simulink model "SistemaCompleto_PMSM"  (R2023b)
settings: Solver=VariableStepAuto  StartTime=0.0  StopTime=2  RelTol=1e-3
PostLoadFcn:
  | parametros_sistema_completo
  | run("parametros_sistema_completo.mlx")
values from neighbouring files (symbols this model uses):
  a_cu = 3.9e-3    (= 0.0039)    [parametros_sistema_completo.m]    (also in workspace_params.mat)
  A_i = [0,  1,                          0 ... (first row only)    [analisis_estabilidad_LA.m]
  b_eq = params.b_total    [calcular_matriz_AO.m]    (also in calculo_incertidumbre_y_control.m = b_m + b_l/(r^2); parametros_sistema_completo.m = 2.19444444444e-05; workspace_params.mat = 2.19444444444e-05)
  C_ts = C_ts * (1 + tol_pct)    [calculo_incertidumbre_y_control.m]    (also in parametros_sistema_completo.m = 0.818; workspace_params.mat = 0.818)
  g = 9.80665    [parametros_sistema_completo.m]    (also in workspace_params.mat)
  J_eq = params.J_total    [calcular_matriz_AO.m]    (also in calculo_incertidumbre_y_control.m = J_m + J_l/r^2; parametros_sistema_completo.m = 1.97847222222e-05; workspace_params.mat = 3.28055555556e-05)
  k_l = m*l_cm + m_l*l_l    [calculo_incertidumbre_y_control.m]    (also in parametros_sistema_completo.m = 0.25; workspace_params.mat = 0.625)
  L_d = L_d    * (1 - tol_pct)    [calculo_incertidumbre_y_control.m]    (also in parametros_sistema_completo.m = 0.0066; workspace_params.mat = 0.0066)
  L_ls = L_ls   * (1 - tol_pct)    [calculo_incertidumbre_y_control.m]    (also in parametros_sistema_completo.m = 0.0008; workspace_params.mat = 0.0008)
  L_q = L_q    * (1 - tol_pct)    [calculo_incertidumbre_y_control.m]    (also in parametros_sistema_completo.m = 0.0058; workspace_params.mat = 0.0058)
  lambda_r = lambda_r * (1 + tol_pct)    [calculo_incertidumbre_y_control.m]    (also in parametros_sistema_completo.m = 0.016; workspace_params.mat = 0.016)
  P_p = 3    [parametros_sistema_completo.m]    (also in workspace_params.mat)
  params = struct()    [evaluar_migracion_Ids.m]    (also in parametros_sistema_completo.m; workspace_params.mat = )
  r = params.r_red    [calcular_matriz_AO.m]    (also in parametros_sistema_completo.m = 120; workspace_params.mat = 120)
  R_s_sim = R_sREF * (1 + a_cu * (T_s_sim - T_sREF))    [configurar_temperatura_516.m]
  R_sREF = R_sREF * (1 - tol_pct)    [calculo_incertidumbre_y_control.m]    (also in parametros_sistema_completo.m = 1.02; workspace_params.mat = 1.02)
  R_ts_amb = R_ts_amb * (1 - tol_pct)    [calculo_incertidumbre_y_control.m]    (also in parametros_sistema_completo.m = 146.7; workspace_params.mat = 146.7)
  T_amb = 20    [parametros_sistema_completo.m]    (also in workspace_params.mat)
  T_s = x(6)    [modulador_torque_521.m]    (also in simulacion_dinamica_516.m)
  T_sREF = 20    [parametros_sistema_completo.m]    (also in workspace_params.mat)
undefined symbols (not defined in the file or in its folder): A_T, A_theta, A_v, b_a, B_i, B_T, B_theta, B_v, C_i, C_T, C_theta, C_v, consigna_posicion, D_i, D_T, D_theta, D_v, i_ds_inicial, Is_pico, Is_rms_max, Is_rms_nom, K_e_i_m_int, K_e_tita_m, K_e_tita_m_int, K_e_w_m, K_e_w_m_int, K_p0, K_pd, K_pq, K_sa, K_sia, pos_inicial, t_rampa_acel, t_rampa_vel, V_sl_max, x0_ias, x0_ibs, x0_ics, x0_T, x0_theta
libraries: simulink_extras x8, SignalEditorBlockLib x6, eeStairGenerator x4, simulink x1
(part 1 of 7)
settings Model: Creator=Francisco  LastModifiedBy=calde
settings DebuggingCC: UnderspecifiedInitializationDetection=Classic  MergeDetectMultiDrivingBlocksExec=none
settings ModelReferenceCC: PropagateSignalLabelsOutOfModel=off

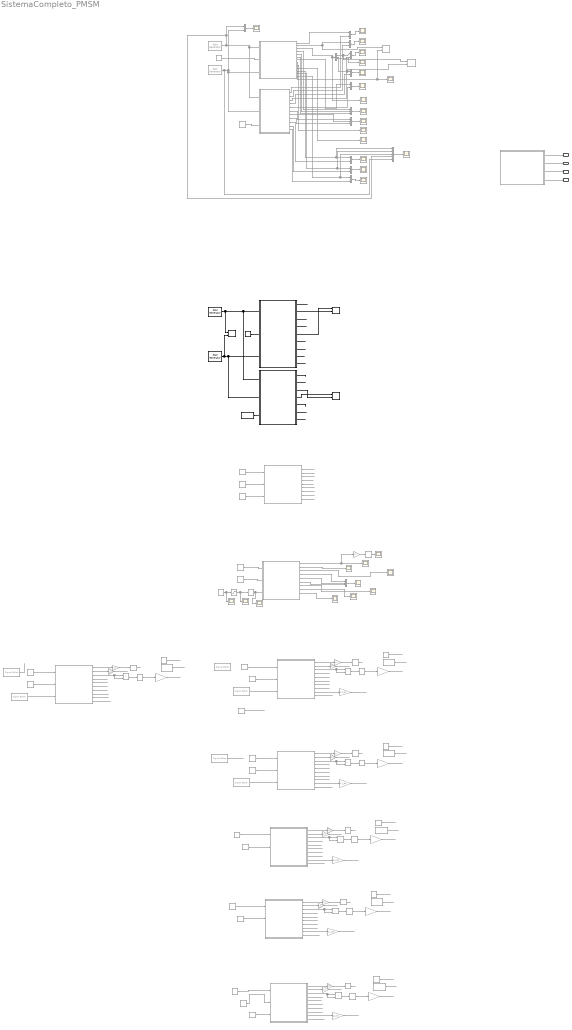
== system SistemaCompleto_PMSM ==
  note: Modelo NL vs LTI Equivalente Aumentado
  note: Consigna de Torque
  note: Consigna de Corriente en eje directo
  note: Consigna de Corriente en eje directo
  note: Consigna de Corriente en eje directo
  note: 5.1.6 Modelo Gobal NL Retroalimentado
      | vs LTI Equivalente Aumentado
  note: Consigna de Corriente en eje directo
  note: Observador de velocidad
      | perfil trapezoidal de velocidad
  note: Consigna de Corriente en eje directo
  note: Consigna de Corriente en eje directo
  note: Consigna de Corriente en eje directo
  note: Consigna de Corriente en eje directo
  note: 5.2.1 Modulador de Torque equivalente
  note: 5.2.2 Controlador externo de movimientos: posición/velocidad
  note: 5.2.3 Observador de velocidad perfil trapezoidal aceleracion
  note: 5.2.7 Controlador Codifiado
  note: 5.2.6 Controlador Discretizado
  note: 5.2.5 Sensores y Acondicionadores de Señal
  note: 5.2.3 Observador de velocidad con accion integral
  Constant{,1..4,6,10..11,14,17,19,23,27} (13 alike) : Constant  Commented=on  Value=0
  Constant{8,12,15,21,25,29} (6 alike) : Constant  Commented=on  Value=Is_rms_max
  Constant{9,13,16,22,26,30} (6 alike) : Constant  Commented=on  Value=Is_rms_nom
  Constant18 : Constant  Commented=on  Value=115
  Constant{7,20,24,28} (4 alike) : Constant  Commented=on  Value=5
  Constant31 : Constant  Commented=on  Value=0.1
  Constant32 : Constant  Commented=on  Value=9.81
  Constant5 : Constant  Value=0
  Degrees to Radians : simulink_extras/Transformations/Degrees to Radians  Commented=on
  Demux : Demux  Commented=on  Outputs=3
  Dot Product{,1..5} (6 alike) : DotProduct  Commented=on  OutDataTypeStr=Inherit: Inherit via internal rule
  Gain{,1,3,5,7,9,11..12,14,16,18,20,22} (13 alike) : Gain  Commented=on  Gain=1/r
  Gain{2,6,10,13,17,21} (6 alike) : Gain  Commented=on  Gain=1/sqrt(2)
  Gain{4,8,15,19,23} (5 alike) : Gain  Commented=on  Gain=1/J_eq
  I_abc : Scope  Commented=on
  I_abc2 : Scope  Commented=on
  I_abc3 : Scope  Commented=on
  I_qds : Scope  Commented=on
  I_qds2 : Scope  Commented=on
  LTI Equivalente Aumentado : Subsystem  Commented=on
  LTI Equivalente Aumentado2 : Subsystem
  LTI Equivalente Nominal : Subsystem  Commented=on
  "Modelo Global " : Subsystem  Commented=on
  Modelo Global NL Controlador modulador de torque : Subsystem  Commented=on
  Modelo Global NL Controlador modulador de torque1 : Subsystem  Commented=on
  Modelo Global NL Controlador modulador de torque3 : Subsystem  Commented=on
  Modelo Global NL Controlador modulador de torque4 : Subsystem  Commented=on
  Modelo Global NL perfil trapezoidal aceleracion : Subsystem  Commented=on
  Modelo Global NL perfil trapezoidal aceleracion y codificado : Subsystem  Commented=on
  Modelo Global NL perfil trapezoidal aceleracion1 : Subsystem  Commented=on
  Modelo Global NL perfil trapezoidal aceleracion2 : Subsystem  Commented=on
  Modelo Global NL Retroalimentado : Subsystem
  Mux{,1..5,8..10} (9 alike) : Mux  Commented=on  Inputs=2
  Mux11 : Mux  Commented=on  Inputs=3
  Mux12 : Mux  Commented=on  Inputs=5
  Mux13 : Mux  Commented=on  Inputs=3
  Mux6 : Mux  Commented=on  Inputs=3
  Radians to Degrees{,1..6} (7 alike) : simulink_extras/Transformations/Radians to Degrees  Commented=on
  Ramp : simulink/Sources/Ramp  Commented=on  slope=300  start=0  InitialOutput=0
  Saturation : Saturate  Commented=on  UpperLimit=135  LowerLimit=0
  Scope1 : Scope  Commented=on
  Scope2 : Scope  Commented=on
  Scope3 : Scope  Commented=on
  Signal Editor : SignalEditorBlockLib/Signal Editor  Commented=on  FileName=C:\Users\calde\OneDrive\Documents\00_INGENIERIA\1_CURSADO\2 2025\AyME\modelado-control-motor-pmsm\Señales y Escenarios\trap_posicion_1.mat  ActiveScenario=TrapezoidalPosicion  ActiveSignal=posicion  IsBus=off  OutputBusObjectStr=Bus: BusObject  SampleTime=0  ZeroCross=off  OutputAfterFinalValue=Setting to zero  Unit=inherit  PreserveSignalName=on  ApplySigPropsToAllScenarios=on  ApplySigPropsToAllSignals=off
  Signal Editor1 : SignalEditorBlockLib/Signal Editor  Commented=on  FileName=C:\Users\calde\OneDrive\Documents\00_INGENIERIA\1_CURSADO\2 2025\AyME\modelado-control-motor-pmsm\Señales\perturbacion_Tld.mat  ActiveScenario=Perturbacion  ActiveSignal=Signal 1  IsBus=off  OutputBusObjectStr=Bus: BusObject  SampleTime=0  Interpolate=off  ZeroCross=off  OutputAfterFinalValue=Setting to zero  Unit=inherit  PreserveSignalName=on  ApplySigPropsToAllScenarios=on  ApplySigPropsToAllSignals=off
  Signal Editor2 : SignalEditorBlockLib/Signal Editor  Commented=on  FileName=D:\05.Estudios\Trabajo Final AyME 2025\modelado-control-motor-pmsm\Señales y Escenarios\trap_posicion_1.mat  ActiveScenario=TrapezoidalPosicion  ActiveSignal=posicion  IsBus=off  OutputBusObjectStr=Bus: BusObject  SampleTime=0  ZeroCross=off  OutputAfterFinalValue=Setting to zero  Unit=inherit  PreserveSignalName=on  ApplySigPropsToAllScenarios=on  ApplySigPropsToAllSignals=off
  Signal Editor3 : SignalEditorBlockLib/Signal Editor  Commented=on  FileName=D:\05.Estudios\Trabajo Final AyME 2025\modelado-control-motor-pmsm\Señales\perturbacion_Tld.mat  ActiveScenario=Perturbacion  ActiveSignal=Signal 1  IsBus=off  OutputBusObjectStr=Bus: BusObject  SampleTime=0  Interpolate=off  ZeroCross=off  OutputAfterFinalValue=Setting to zero  Unit=inherit  PreserveSignalName=on  ApplySigPropsToAllScenarios=on  ApplySigPropsToAllSignals=off
  Signal Editor4 : SignalEditorBlockLib/Signal Editor  Commented=on  FileName=D:\05.Estudios\Trabajo Final AyME 2025\modelado-control-motor-pmsm\Señales y Escenarios\trap_posicion_1.mat  ActiveScenario=TrapezoidalPosicion  ActiveSignal=posicion  IsBus=off  OutputBusObjectStr=Bus: BusObject  SampleTime=0  ZeroCross=off  OutputAfterFinalValue=Setting to zero  Unit=inherit  PreserveSignalName=on  ApplySigPropsToAllScenarios=on  ApplySigPropsToAllSignals=off
  Signal Editor5 : SignalEditorBlockLib/Signal Editor  Commented=on  FileName=D:\05.Estudios\Trabajo Final AyME 2025\modelado-control-motor-pmsm\Señales\perturbacion_Tld.mat  ActiveScenario=Perturbacion  ActiveSignal=Signal 1  IsBus=off  OutputBusObjectStr=Bus: BusObject  SampleTime=0  Interpolate=off  ZeroCross=off  OutputAfterFinalValue=Setting to zero  Unit=inherit  PreserveSignalName=on  ApplySigPropsToAllScenarios=on  ApplySigPropsToAllSignals=off
  Sqrt{,1..5} (6 alike) : Sqrt  Commented=on
  T_amb : Constant  Commented=on  Value=T_amb
  T_amb2 : Constant  Value=T_amb
  T_l : eeStairGenerator/Stair Generator  Commented=on  LabelModeActiveChoice=Discrete  TimeInput=[0 0.3 0.5 0.9 1.3 1.5 1.9]  AmplitudeInput=[0 6.28 -6.28 0 6.28 -6.28 0]  SampleTime=1e-3  RepeatPattern=off  OutDataTypeStr=double
      settings: LibrarySourceBlock=ee_sl_lib/General Control/Stair Generator
  T_l2 : eeStairGenerator/Stair Generator  LabelModeActiveChoice=Discrete  TimeInput=[0 0.3 0.5 0.9 1.3 1.5 1.9]  AmplitudeInput=[0 6.28 -6.28 0 6.28 -6.28 0]  SampleTime=1e-3  RepeatPattern=off  OutDataTypeStr=double
      settings: LibrarySourceBlock=ee_sl_lib/General Control/Stair Generator
  T_m [N.m] : Scope  Commented=on
  T_m [N.m]3 : Scope  Commented=on
  T_m [N.m]4 : Scope  Commented=on
  T_s (vs) : Scope  Commented=on
  T_s(t)1 : Scope  Commented=on
  Torque vs. Velocidad : Record  Commented=on  FileSettingsInternal="{\"entries\":[{\"content\":{\"excelSettings\":{\"content\":{},\"type\":\"Streamout.ExcelSettings\"}},\"type\":\"Streamout.FileSettingStorage\",\"uuid\":\"\"}],\"packageUris\":[\"http:\\/\\/schema.mathworks.com\\/mf0\\/streamout_blocks\\/R2020a\"],\"version\":\"1.0\"}"  Layout=[1 1]  SignalsInternal="{\"entries\":[{\"content\":{},\"type\":\"RecordBlkView.InputSignals\",\"uuid\":\"\"}],\"packageUris\":[\"http:\\/\\/schema.mathworks.com\\/mf0\\/streamout_blocks\\/R2020a\"],\"version\":\"1.0\"}"  VisualizationBindings="{\"xyplotplugin\":{\"info\":[{\"series\":[],\"subplotID\":1}]}}"  CompatibilityTag=XY
  Torque vs. Velocidad2 : Record  FileSettingsInternal="{\"entries\":[{\"content\":{\"excelSettings\":{\"content\":{},\"type\":\"Streamout.ExcelSettings\"}},\"type\":\"Streamout.FileSettingStorage\",\"uuid\":\"\"}],\"packageUris\":[\"http:\\/\\/schema.mathworks.com\\/mf0\\/streamout_blocks\\/R2020a\"],\"version\":\"1.0\"}"  Layout=[1 1]  SignalsInternal="{\"entries\":[{\"content\":{\"signals\":[{\"content\":{\"blockPath\":[],\"dimensions\":[1],\"domain\":\"\",\"lineColor\":\"#d95319\",\"port\":1,\"sid\":[\"\"],\"signalID\":4289,\"signalName\":\"NL T_m [N.m]\"},\"type\":\"RecordBlkView.Signal\",\"uuid\":\"\"},{\"content\":{\"blockPath\":[],\"dimensions\":[1],\"domain\":\"\",\"lineColor\":\"#edb120\",\"port\":2,\"sid\":[\"\"],\"signalID\":4293,\"signalName\":\"NL ω_m [rad\\/s]\"},\"type\":\"RecordBlkView.Signal\",\"uuid\":\"\"}]},\"type\":\"RecordBlkView.InputSignals\",\"uuid\":\"\"}],\"packageUris\":[\"http:\\/\\/schema.mathworks.com\\/mf0\\/streamout_blocks\\/R2020a\"],\"version\":\"1.0\"}"  VisualizationBindings="{\"xyplotplugin\":{\"info\":[{\"series\":[],\"subplotID\":1}]}}"  CompatibilityTag=XY
  V_a : Scope  Commented=on
  V_abc vs V_qs-T_l : Scope  Commented=on
  V_b : Scope  Commented=on
  V_c : Scope  Commented=on
  V_ds : Scope  Commented=on
  V_qs* : eeStairGenerator/Stair Generator  Commented=on  LabelModeActiveChoice=Discrete  TimeInput=[0 0.1 0.7 1.1 1.7]  AmplitudeInput=[0 19.596 0 -19.596 0]  SampleTime=1e-3  RepeatPattern=off  OutDataTypeStr=double
      settings: LibrarySourceBlock=ee_sl_lib/General Control/Stair Generator
  V_qs*2 : eeStairGenerator/Stair Generator  LabelModeActiveChoice=Discrete  TimeInput=[0 0.1 0.7 1.1 1.7]  AmplitudeInput=[0 19.596 0 -19.596 0]  SampleTime=1e-3  RepeatPattern=off  OutDataTypeStr=double
      settings: LibrarySourceBlock=ee_sl_lib/General Control/Stair Generator
  "V_qs, T_l vs t" : Scope  Commented=on
  "V_qs, T_l vs t2" : Record  FileSettingsInternal="{\"entries\":[{\"content\":{\"excelSettings\":{\"content\":{},\"type\":\"Streamout.ExcelSettings\"}},\"type\":\"Streamout.FileSettingStorage\",\"uuid\":\"\"}],\"packageUris\":[\"http:\\/\\/schema.mathworks.com\\/mf0\\/streamout_blocks\\/R2020a\"],\"version\":\"1.0\"}"  Layout=[1 1]  SignalsInternal="{\"entries\":[{\"content\":{\"signals\":[{\"content\":{\"blockPath\":[],\"dimensions\":[1,1],\"domain\":\"\",\"lineColor\":\"#b746ff\",\"lineWidth\":2,\"port\":1,\"sid\":[\"\"],\"signalID\":4297,\"signalName\":\"V_qs*\"},\"type\":\"RecordBlkView.Signal\",\"uuid\":\"\"},{\"content\":{\"blockPath\":[],\"dimensions\":[1,1],\"domain\":\"\",\"lineColor\":\"#64d413\",\"lineWidth\":2,\"port\":2,\"sid\":[\"\"],\"signalID\":4301,\"signalName\":\"T_l\"},\"type\":\"RecordBlkView.Signal\",\"uuid\":\"\"}]},\"type\":\"RecordBlkView.InputSignals\",\"uuid\":\"\"}],\"packageUris\":[\"http:\\/\\/schema.mathworks.com\\/mf0\\/streamout_blocks\\/R2020a\"],\"version\":\"1.0\"}"  VisualizationBindings="{\"xyplotplugin\":{\"info\":[{\"series\":[],\"subplotID\":1}]}}"  CompatibilityTag=XY
  i_0s vs t : Scope  Commented=on
  i_ds vs i_qs : Record  Commented=on  FileSettingsInternal="{\"entries\":[{\"content\":{\"excelSettings\":{\"content\":{},\"type\":\"Streamout.ExcelSettings\"}},\"type\":\"Streamout.FileSettingStorage\",\"uuid\":\"\"}],\"packageUris\":[\"http:\\/\\/schema.mathworks.com\\/mf0\\/streamout_blocks\\/R2020a\"],\"version\":\"1.0\"}"  Layout=[1 1]  SignalsInternal="{\"entries\":[{\"content\":{},\"type\":\"RecordBlkView.InputSignals\",\"uuid\":\"\"}],\"packageUris\":[\"http:\\/\\/schema.mathworks.com\\/mf0\\/streamout_blocks\\/R2020a\"],\"version\":\"1.0\"}"  VisualizationBindings="{\"xyplotplugin\":{\"info\":[{\"series\":[],\"subplotID\":1}]}}"  CompatibilityTag=XY
  i_ds vs i_qs2 : Record  FileSettingsInternal="{\"entries\":[{\"content\":{\"excelSettings\":{\"content\":{},\"type\":\"Streamout.ExcelSettings\"}},\"type\":\"Streamout.FileSettingStorage\",\"uuid\":\"\"}],\"packageUris\":[\"http:\\/\\/schema.mathworks.com\\/mf0\\/streamout_blocks\\/R2020a\"],\"version\":\"1.0\"}"  Layout=[1 1]  SignalsInternal="{\"entries\":[{\"content\":{\"signals\":[{\"content\":{\"blockPath\":[],\"dimensions\":[1],\"domain\":\"\",\"lineColor\":\"#4dbeee\",\"port\":1,\"sid\":[\"\"],\"signalID\":4305,\"signalName\":\"LTI i_ds [A\"},\"type\":\"RecordBlkView.Signal\",\"uuid\":\"\"},{\"content\":{\"blockPath\":[],\"dimensions\":[1],\"domain\":\"\",\"lineColor\":\"#a2142f\",\"port\":2,\"sid\":[\"\"],\"signalID\":4309,\"signalName\":\"LTI i_qs [A]\"},\"type\":\"RecordBlkView.Signal\",\"uuid\":\"\"}]},\"type\":\"RecordBlkView.InputSignals\",\"uuid\":\"\"}],\"packageUris\":[\"http:\\/\\/schema.mathworks.com\\/mf0\\/streamout_blocks\\/R2020a\"],\"version\":\"1.0\"}"  VisualizationBindings="{\"xyplotplugin\":{\"info\":[{\"series\":[],\"subplotID\":1}]}}"  CompatibilityTag=XY
  i_ds vs t : Scope  Commented=on
  i_qs vs t : Scope  Commented=on
  δ [rad] : Scope  Commented=on
  θm(t) vs t : Scope  Commented=on
  θm(t) vs t 2 : Scope  Commented=on
  θm(t) vs t 3 : Scope  Commented=on
  ωm(t) vs t : Scope  Commented=on
  ωm(t) vs t2 : Scope  Commented=on
  θ_m : Outport
  ω_m : Outport  Port=2
  i_qs : Outport  Port=3
  T_s : Outport  Port=4
  wires:
  LTI Equivalente Nominal/1(θ_m) -> θ_m/1
  LTI Equivalente Nominal/2(ω_m) -> ω_m/1
  LTI Equivalente Nominal/3(i_qs) -> i_qs/1
  LTI Equivalente Nominal/4(T_s) -> T_s/1
  V_qs*/1 -> Mux12/4, Mux5/1, LTI Equivalente Aumentado/1(v_qs), "Modelo Global "/1(V_qs*[V])
  T_l/1 -> Mux12/5, LTI Equivalente Aumentado/2(T_ld), "Modelo Global "/3(Tld [N.m]), Mux5/2
  T_amb/1 -> LTI Equivalente Aumentado/3(T_amb)
  Constant/1 -> "Modelo Global "/2(V_ds*[V])
  LTI Equivalente Aumentado/1(θ_m [rad]) -> Mux/2
  Mux/1 -> θm(t) vs t/1
  "Modelo Global "/1(θ_m [rad]) -> Mux/1
  "Modelo Global "/3(I_qd0s [A]) -> I_qds/1, Demux/1
  Demux/1 -> Mux3/1, i_ds vs i_qs/1
  Demux/2 -> i_ds vs i_qs/2, Mux2/1
  LTI Equivalente Aumentado/3(i_qs [A]) -> Mux3/2
  LTI Equivalente Aumentado/4(i_ds [A]) -> Mux2/2
  Mux3/1 -> i_qs vs t/1
  Mux2/1 -> i_ds vs t/1
  "Modelo Global "/7(T_s [°C]) -> Mux1/1
  LTI Equivalente Aumentado/5(T_s [°C]) -> Mux1/2
  Mux1/1 -> T_s (vs)/1
  Mux4/1 -> ωm(t) vs t/1
  "Modelo Global "/2(ω_m [rad/s]) -> Mux4/1, Torque vs. Velocidad/1  "ω_m [rad/s]"
  LTI Equivalente Aumentado/2(ω_m [rad/s]) -> Mux4/2
  "Modelo Global "/8(T_m [N.m]) -> Torque vs. Velocidad/2, T_m [N.m]/1  "T_m [N.m]"
  Mux5/1 -> "V_qs, T_l vs t"/1
  Mux6/1 -> I_abc/1
  "Modelo Global "/4(I_a [A]) -> Mux6/1
  "Modelo Global "/5(I_b [A]) -> Mux6/2
  "Modelo Global "/6(I_c [A]) -> Mux6/3
  Demux/3 -> i_0s vs t/1
  "Modelo Global "/9(δ [rad]) -> δ [rad]/1  "δ [rad]"
  "Modelo Global "/10(V_ds[V]) -> V_ds/1
  Mux10/1 -> V_c/1
  Mux9/1 -> V_b/1
  Mux8/1 -> V_a/1
  LTI Equivalente Aumentado/9(V_a) -> Mux8/2
  LTI Equivalente Aumentado/10(V_b) -> Mux9/2
  LTI Equivalente Aumentado/11(V_c) -> Mux10/2
  "Modelo Global "/11(V_a) -> Mux12/1, Mux8/1
  "Modelo Global "/12(V_b) -> Mux12/2, Mux9/1
  "Modelo Global "/13(V_c) -> Mux12/3, Mux10/1
  Mux11/1 -> I_abc2/1
  LTI Equivalente Aumentado/6(I_a [A]) -> Mux11/1
  LTI Equivalente Aumentado/7(I_b [A]) -> Mux11/2
  LTI Equivalente Aumentado/8(I_c [A]) -> Mux11/3
  Mux12/1 -> V_abc vs V_qs-T_l/1
  Modelo Global NL Controlador modulador de torque/5(I_b [A]) -> ?  "I_b [A]"
  Modelo Global NL Controlador modulador de torque/3(I_qd0s [A]) -> ?  "I_qd0s [A]"
  Constant2/1 -> Modelo Global NL Controlador modulador de torque/2(i_ds*)
  Modelo Global NL Controlador modulador de torque/6(I_c [A]) -> ?  "I_c [A]"
  Modelo Global NL Controlador modulador de torque/7(T_s [°C]) -> ?  "T_s [°C]"
  Modelo Global NL Controlador modulador de torque/1(θm(t) [rad]) -> ?  "θm(t) [rad]"
  Modelo Global NL Controlador modulador de torque/4(I_a [A]) -> ?  "I_a [A]"
  Constant1/1 -> Modelo Global NL Controlador modulador de torque/1(Tld [N.m])
  Modelo Global NL Controlador modulador de torque/2(ωm(t) [rad/s]) -> ?  "ωm(t) [rad/s]"
  Modelo Global NL Controlador modulador de torque/8(T_m [N.m]) -> ?  "T_m [N.m]"
  Constant31/1 -> Modelo Global NL Controlador modulador de torque/3(T_m*[N.m])  "T_m*[N.m]"
  Modelo Global NL Controlador modulador de torque1/8(T_m [N.m]) -> T_m [N.m]3/1  "T_m [N.m]"
  Modelo Global NL Controlador modulador de torque1/4(I_a [A]) -> Mux13/1
  Modelo Global NL Controlador modulador de torque1/3(I_qd0s [A]) -> I_qds2/1
  Modelo Global NL Controlador modulador de torque1/6(I_c [A]) -> Mux13/3
  Modelo Global NL Controlador modulador de torque1/1(θm(t) [rad]) -> Gain/1, θm(t) vs t 2/1  "θm(t) [rad]"
  Constant4/1 -> Modelo Global NL Controlador modulador de torque1/2(i_ds*)
  Modelo Global NL Controlador modulador de torque1/5(I_b [A]) -> Mux13/2
  Modelo Global NL Controlador modulador de torque1/2(ωm(t) [rad/s]) -> ωm(t) vs t2/1  "ωm(t) [rad/s]"
  Constant3/1 -> Modelo Global NL Controlador modulador de torque1/1(Tld [N.m])
  Mux13/1 -> I_abc3/1
  Modelo Global NL Controlador modulador de torque1/7(T_s [°C]) -> T_s(t)1/1
  Degrees to Radians/1 -> Scope3/1, Modelo Global NL Controlador modulador de torque1/3(θl*(t))
  Saturation/1 -> Scope1/1, Degrees to Radians/1
  Ramp/1 -> Scope2/1, Saturation/1
  Gain/1 -> Radians to Degrees/1
  Radians to Degrees/1 -> θm(t) vs t 3/1
  Modelo Global NL Controlador modulador de torque1/9(T_neto) -> T_m [N.m]4/1  "T_neto [N.m]"
  Radians to Degrees1/1 -> ?
  Modelo Global NL perfil trapezoidal aceleracion/4(I_a [A]) -> ?  "I_a [A]"
  Modelo Global NL perfil trapezoidal aceleracion/9(T_neto) -> Gain4/1  "T_neto [N.m]"
  Modelo Global NL perfil trapezoidal aceleracion/1(θm(t) [rad]) -> Gain1/1  "θm(t) [rad]"
  Gain1/1 -> Radians to Degrees1/1  "θl(t) [rad]"
  Modelo Global NL perfil trapezoidal aceleracion/5(I_b [A]) -> ?  "I_b [A]"
  Modelo Global NL perfil trapezoidal aceleracion/6(I_c [A]) -> ?  "I_c [A]"
  Modelo Global NL perfil trapezoidal aceleracion/7(T_s [°C]) -> ?  "T_s [°C]"
  Constant6/1 -> Modelo Global NL perfil trapezoidal aceleracion/2(i_ds*)
  Modelo Global NL perfil trapezoidal aceleracion/2(ω~_m(t) [rad/s]) -> Gain3/1  "ω~_m(t) [rad/s]"
  Modelo Global NL perfil trapezoidal aceleracion/8(T_m [N.m]) -> ?  "T_m [N.m]"
  Signal Editor/1 -> Modelo Global NL perfil trapezoidal aceleracion/3(θl*(t))  "θl*(t) [rad]"
  Gain2/1 -> ?  "I_rms"
  Modelo Global NL perfil trapezoidal aceleracion/3(I_qd0s [A]) -> Dot Product/2, Dot Product/1  "I_qd0s [A]"
  Dot Product/1 -> Sqrt/1
  Sqrt/1 -> Gain2/1  "I_stator"
  Constant8/1 -> ?  "I_rms_max"
  Constant9/1 -> ?  "I_rms_nom"
  Modelo Global NL Retroalimentado/3(I_qd0s [A]) -> ?  "NL I_qd0s [A]"
  Modelo Global NL Retroalimentado/1(θ_m [rad]) -> ?  "NL θ_m [rad]"
  LTI Equivalente Aumentado2/1(θ_m [rad]) -> ?  "LTI θ_m [rad]"
  Modelo Global NL Retroalimentado/4(T_s [°C]) -> ?  "NL T_s [°C]"
  Modelo Global NL Retroalimentado/6(δ [deg]) -> ?  "NL δ [deg]"
  Modelo Global NL Retroalimentado/7(V_ds[V]) -> ?  "NL V_ds[V]"
  Modelo Global NL Retroalimentado/9(V_abc [V]) -> ?  "NL V_abc [V]"
  LTI Equivalente Aumentado2/6(I_abc [A]) -> ?  "LTI I_abc [A]"
  Modelo Global NL Retroalimentado/8(I_abc [A]) -> ?  "NL I_abc [A]"
  LTI Equivalente Aumentado2/7(V_abc [V]) -> ?  "LTI V_abc [V]"
  LTI Equivalente Aumentado2/5(T_s [°C]) -> ?  "LTI T_s [°C]"
  LTI Equivalente Aumentado2/4(i_ds [A]) -> i_ds vs i_qs2/1  "LTI i_ds [A"
  T_l2/1 -> Modelo Global NL Retroalimentado/3(Tld [N.m]), LTI Equivalente Aumentado2/2(T_ld), "V_qs, T_l vs t2"/2  "T_l"
  Constant5/1 -> Modelo Global NL Retroalimentado/2(V_ds*[V])  "v_ds*"
  LTI Equivalente Aumentado2/3(i_qs [A]) -> i_ds vs i_qs2/2  "LTI i_qs [A]"
  LTI Equivalente Aumentado2/2(ω_m [rad/s]) -> ?  "LTI ω_m [rad/s]"
  V_qs*2/1 -> Modelo Global NL Retroalimentado/1(V_qs*[V]), LTI Equivalente Aumentado2/1(v_qs), "V_qs, T_l vs t2"/1  "V_qs*"
  Modelo Global NL Retroalimentado/2(ω_m [rad/s]) -> Torque vs. Velocidad2/2  "NL ω_m [rad/s]"
  T_amb2/1 -> LTI Equivalente Aumentado2/3(T_amb)
  Modelo Global NL Retroalimentado/5(T_m [N.m]) -> Torque vs. Velocidad2/1  "NL T_m [N.m]"
  Constant7/1 -> Modelo Global NL perfil trapezoidal aceleracion/1(Tld [N.m])  "Tld [N.m]"
  Gain3/1 -> ?  "ω~_l(t) [rad/s]"
  Modelo Global NL perfil trapezoidal aceleracion/10(θl* [rad]) -> ?  "Trayectoria Pos"
  Gain4/1 -> ?  "Aceleracion"
  Signal Editor3/1 -> ?  "Tld [N.m]"
  Gain8/1 -> ?  "Aceleracion"
  Sqrt1/1 -> Gain6/1  "I_stator"
  Modelo Global NL Controlador modulador de torque3/2(ω~_m(t) [rad/s]) -> Gain7/1  "ω~_m(t) [rad/s]"
  Dot Product1/1 -> Sqrt1/1
  Modelo Global NL Controlador modulador de torque3/1(θm(t) [rad]) -> Gain5/1  "θm(t) [rad]"
  Gain5/1 -> Radians to Degrees2/1  "θl(t) [rad]"
  Constant11/1 -> Modelo Global NL Controlador modulador de torque3/1(Tld [N.m])
  Modelo Global NL Controlador modulador de torque3/9(T_neto) -> Gain8/1  "T_neto [N.m]"
  Modelo Global NL Controlador modulador de torque3/3(I_qd0s [A]) -> Dot Product1/2, Dot Product1/1  "I_qd0s [A]"
  Gain7/1 -> ?  "ω~_l(t) [rad/s]"
  Signal Editor2/1 -> Modelo Global NL Controlador modulador de torque3/3(θl*(t))  "θl*(t) [rad]"
  Constant10/1 -> Modelo Global NL Controlador modulador de torque3/2(i_ds*)
  Radians to Degrees2/1 -> ?
  Modelo Global NL Controlador modulador de torque3/4(I_a [A]) -> ?  "I_a [A]"
  Modelo Global NL Controlador modulador de torque3/8(T_m [N.m]) -> ?  "T_m [N.m]"
  Gain6/1 -> ?  "I_rms"
  Constant12/1 -> ?  "I_rms_max"
  Modelo Global NL Controlador modulador de torque3/5(I_b [A]) -> ?  "I_b [A]"
  Modelo Global NL Controlador modulador de torque3/6(I_c [A]) -> ?  "I_c [A]"
  Modelo Global NL Controlador modulador de torque3/10(θl* [rad]) -> ?  "Trayectoria Pos"
  Modelo Global NL Controlador modulador de torque3/7(T_s [°C]) -> ?  "T_s [°C]"
  Constant13/1 -> ?  "I_rms_nom"
  Gain9/1 -> Radians to Degrees3/1  "θl(t) [rad]"
  Modelo Global NL Controlador modulador de torque4/4(I_a [A]) -> ?  "I_a [A]"
  Modelo Global NL Controlador modulador de torque4/5(I_b [A]) -> ?  "I_b [A]"
  Radians to Degrees3/1 -> ?
  Modelo Global NL Controlador modulador de torque4/6(I_c [A]) -> ?  "I_c [A]"
  Modelo Global NL Controlador modulador de torque4/8(T_m [N.m]) -> ?  "T_m [N.m]"
  Modelo Global NL Controlador modulador de torque4/7(T_s [°C]) -> ?  "T_s [°C]"
  Constant15/1 -> ?  "I_rms_max"
  Constant16/1 -> ?  "I_rms_nom"
  Gain11/1 -> ?  "ω~_l(t) [rad/s]"
  Modelo Global NL Controlador modulador de torque4/10(θm* [rad]) -> ?  "Trayectoria Pos"
  Modelo Global NL Controlador modulador de torque4/3(I_qd0s [A]) -> Dot Product2/2, Dot Product2/1  "I_qd0s [A]"
  Sqrt2/1 -> Gain10/1  "I_stator"
  Signal Editor4/1 -> Modelo Global NL Controlador modulador de torque4/3(θl*(t))  "θl*(t) [rad]"
  Dot Product2/1 -> Sqrt2/1
  Gain10/1 -> ?  "I_rms"
  Signal Editor5/1 -> ?  "Tld [N.m]"
  Constant14/1 -> Modelo Global NL Controlador modulador de torque4/2(i_ds*)
  Modelo Global NL Controlador modulador de torque4/9(T_neto) -> ?  "T_neto [N.m]"
  Modelo Global NL Controlador modulador de torque4/2(ω~_m(t) [rad/s]) -> Gain11/1  "ω~_m(t) [rad/s]"
  Modelo Global NL Controlador modulador de torque4/1(θm(t) [rad]) -> Gain9/1  "θm(t) [rad]"
  Constant17/1 -> Modelo Global NL Controlador modulador de torque4/1(Tld [N.m])
  Constant18/1 -> ?  "Ts°_max"
  Constant20/1 -> Modelo Global NL perfil trapezoidal aceleracion1/1(Tld [N.m])  "Tld [N.m]"
  ? -> Modelo Global NL perfil trapezoidal aceleracion1/3(θl*(t))  "θl*(t) [rad]"
  Modelo Global NL perfil trapezoidal aceleracion1/3(I_qd0s [A]) -> Dot Product3/2, Dot Product3/1  "I_qd0s [A]"
  Constant19/1 -> Modelo Global NL perfil trapezoidal aceleracion1/2(i_ds*)
  Modelo Global NL perfil trapezoidal aceleracion1/9(T_neto) -> Gain15/1  "T_neto [N.m]"
  Modelo Global NL perfil trapezoidal aceleracion1/2(ω~_m(t) [rad/s]) -> Gain14/1  "ω~_m(t) [rad/s]"
  Gain15/1 -> ?  "Aceleracion"
  Modelo Global NL perfil trapezoidal aceleracion1/10(θl* [rad]) -> ?  "Trayectoria Pos"
  Gain12/1 -> Radians to Degrees4/1  "θl,med(t) [rad]"
  Dot Product3/1 -> Sqrt3/1
  Gain14/1 -> ?  "ω~_l(t) [rad/s]"
  Modelo Global NL perfil trapezoidal aceleracion1/1(θm(t) [rad]) -> Gain12/1  "θm(t) [rad]"
  Modelo Global NL perfil trapezoidal aceleracion1/6(I_c [A]) -> ?  "I_c [A]"
  Constant22/1 -> ?  "I_rms_nom"
  Modelo Global NL perfil trapezoidal aceleracion1/7(T_s [°C]) -> ?  "T_s [°C]"
  Gain13/1 -> ?  "I_rms"
  Constant21/1 -> ?  "I_rms_max"
  Modelo Global NL perfil trapezoidal aceleracion1/8(T_m [N.m]) -> ?  "T_m [N.m]"
  Sqrt3/1 -> Gain13/1  "I_stator"
  Modelo Global NL perfil trapezoidal aceleracion1/5(I_b [A]) -> ?  "I_b [A]"
  Radians to Degrees4/1 -> ?
  Modelo Global NL perfil trapezoidal aceleracion1/4(I_a [A]) -> ?  "I_a [A]"
  Modelo Global NL perfil trapezoidal aceleracion2/4(I_a [A]) -> ?  "I_a [A]"
  Radians to Degrees5/1 -> ?
  Modelo Global NL perfil trapezoidal aceleracion2/5(I_b [A]) -> ?  "I_b [A]"
  Sqrt4/1 -> Gain17/1  "I_stator"
  Modelo Global NL perfil trapezoidal aceleracion2/8(T_m [N.m]) -> ?  "T_m [N.m]"
  Constant25/1 -> ?  "I_rms_max"
  Gain17/1 -> ?  "I_rms"
  Modelo Global NL perfil trapezoidal aceleracion2/7(T_s [°C]) -> ?  "T_s [°C]"
  Constant26/1 -> ?  "I_rms_nom"
  Modelo Global NL perfil trapezoidal aceleracion2/6(I_c [A]) -> ?  "I_c [A]"
  Modelo Global NL perfil trapezoidal aceleracion2/1(θm(t) [rad]) -> Gain16/1  "θm(t) [rad]"
  Gain18/1 -> ?  "ω~_l(t) [rad/s]"
  Dot Product4/1 -> Sqrt4/1
  Gain16/1 -> Radians to Degrees5/1  "θl,med(t) [rad]"
  Modelo Global NL perfil trapezoidal aceleracion2/10(θl* [rad]) -> ?  "Trayectoria Pos"
  Gain19/1 -> ?  "Aceleracion"
  Modelo Global NL perfil trapezoidal aceleracion2/2(ω~_m(t) [rad/s]) -> Gain18/1  "ω~_m(t) [rad/s]"
  Modelo Global NL perfil trapezoidal aceleracion2/9(T_neto) -> Gain19/1  "T_neto [N.m]"
  Constant23/1 -> Modelo Global NL perfil trapezoidal aceleracion2/2(i_ds*)
  Modelo Global NL perfil trapezoidal aceleracion2/3(I_qd0s [A]) -> Dot Product4/1, Dot Product4/2  "I_qd0s [A]"
  ? -> Modelo Global NL perfil trapezoidal aceleracion2/3(θl*(t))  "θl*(t) [rad]"
  Constant24/1 -> Modelo Global NL perfil trapezoidal aceleracion2/1(Tld [N.m])  "Tld [N.m]"
  Constant28/1 -> Modelo Global NL perfil trapezoidal aceleracion y codificado/1(Tld [N.m])  "Tld [N.m]"
  ? -> ?  "θl*(t) [rad]"
  Modelo Global NL perfil trapezoidal aceleracion y codificado/3(I_qd0s [A]) -> Dot Product5/2, Dot Product5/1  "I_qd0s [A]"
  Constant27/1 -> Modelo Global NL perfil trapezoidal aceleracion y codificado/2(i_ds*)
  Modelo Global NL perfil trapezoidal aceleracion y codificado/9(T_neto) -> Gain23/1  "T_neto [N.m]"
  Modelo Global NL perfil trapezoidal aceleracion y codificado/2(ω~_m(t) [rad/s]) -> Gain22/1  "ω~_m(t) [rad/s]"
  Gain23/1 -> ?  "Aceleracion"
  Modelo Global NL perfil trapezoidal aceleracion y codificado/10(θl* [rad]) -> ?  "Trayectoria Pos"
  Gain20/1 -> Radians to Degrees6/1  "θl,med(t) [rad]"
  Dot Product5/1 -> Sqrt5/1
  Gain22/1 -> ?  "ω~_l(t) [rad/s]"
  Modelo Global NL perfil trapezoidal aceleracion y codificado/1(θm(t) [rad]) -> Gain20/1  "θm(t) [rad]"
  Modelo Global NL perfil trapezoidal aceleracion y codificado/6(I_c [A]) -> ?  "I_c [A]"
  Constant30/1 -> ?  "I_rms_nom"
  Modelo Global NL perfil trapezoidal aceleracion y codificado/7(T_s [°C]) -> ?  "T_s [°C]"
  Gain21/1 -> ?  "I_rms"
  Constant29/1 -> ?  "I_rms_max"
  Modelo Global NL perfil trapezoidal aceleracion y codificado/8(T_m [N.m]) -> ?  "T_m [N.m]"
  Sqrt5/1 -> Gain21/1  "I_stator"
  Modelo Global NL perfil trapezoidal aceleracion y codificado/5(I_b [A]) -> ?  "I_b [A]"
  Radians to Degrees6/1 -> ?
  Modelo Global NL perfil trapezoidal aceleracion y codificado/4(I_a [A]) -> ?  "I_a [A]"
  Modelo Global NL Controlador modulador de torque/9(T_neto) -> ?  "T_neto [N.m]"
  Constant32/1 -> Modelo Global NL perfil trapezoidal aceleracion y codificado/3(g [m/s2])

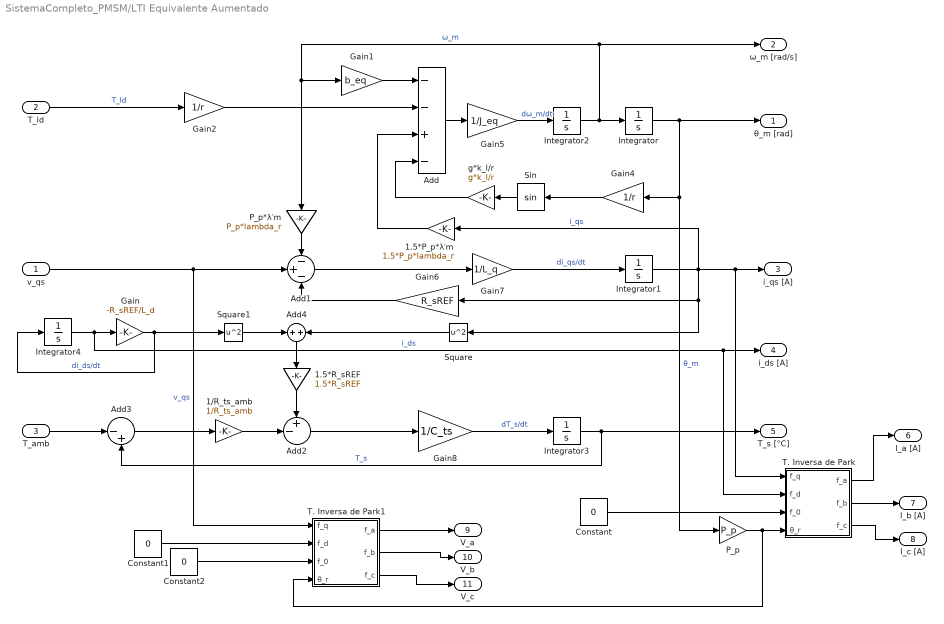
== system SistemaCompleto_PMSM/LTI Equivalente Aumentado ==
  v_qs : Inport
  T_ld : Inport  Port=2
  T_amb : Inport  Port=3
  1.5*P_p*λ′m : Gain  Gain=1.5*P_p*lambda_r
  1.5*R_sREF : Gain  Gain=1.5*R_sREF
  1/R_ts_amb : Gain  Gain=1/R_ts_amb
  Add : Sum  Inputs=--+-
  Add1 : Sum  Inputs=-+-
  Add2 : Sum  Inputs=+-|
  Add3 : Sum  Inputs=|-+
  Add4 : Sum
  Constant : Constant  Value=0
  Constant1 : Constant  Value=0
  Constant2 : Constant  Value=0
  Gain : Gain  Gain=-R_sREF/L_d
  Gain1 : Gain  Gain=b_eq
  Gain2 : Gain  Gain=1/r
  Gain4 : Gain  Gain=1/r
  Gain5 : Gain  Gain=1/J_eq
  Gain6 : Gain  Gain=R_sREF
  Gain7 : Gain  Gain=1/L_q
  Gain8 : Gain  Gain=1/C_ts
  Integrator{,1..2,4} (4 alike) : Integrator
  Integrator3 : Integrator  InitialCondition=T_amb
  P_p : Gain  Gain=P_p
  P_p*λ′m : Gain  Gain=P_p*lambda_r
  Sin : Trigonometry
  Square : Math  Operator=square
  Square1 : Math  Operator=square
  T. Inversa de Park : Subsystem
  T. Inversa de Park1 : Subsystem
  g*k_l/r : Gain  Gain=g*k_l/r
  θ_m [rad] : Outport
  ω_m [rad/s] : Outport  Port=2
  i_qs [A] : Outport  Port=3
  i_ds [A] : Outport  Port=4
  T_s [°C] : Outport  Port=5
  I_a [A] : Outport  Port=6
  I_b [A] : Outport  Port=7
  I_c [A] : Outport  Port=8
  V_a : Outport  Port=9
  V_b : Outport  Port=10
  V_c : Outport  Port=11
  wires:
  P_p*λ′m/1 -> Add1/1
  Add/1 -> Gain5/1
  T_amb/1 -> Add3/1
  g*k_l/r/1 -> Add/4
  Gain1/1 -> Add/1
  v_qs/1 -> T. Inversa de Park1/1(f_q), Add1/2  "v_qs"
  1.5*P_p*λ′m/1 -> Add/3
  Gain6/1 -> Add1/3
  Gain2/1 -> Add/2
  T_ld/1 -> Gain2/1  "T_ld"
  Sin/1 -> g*k_l/r/1
  1.5*R_sREF/1 -> Add2/1
  1/R_ts_amb/1 -> Add2/2
  Add2/1 -> Gain8/1
  Square/1 -> Add4/2
  Gain5/1 -> Integrator2/1  "dω_m/dt"
  Gain4/1 -> Sin/1
  Add3/1 -> 1/R_ts_amb/1
  Integrator3/1 -> T_s [°C]/1, Add3/2  "T_s"
  Gain7/1 -> Integrator1/1  "di_qs/dt"
  Integrator/1 -> P_p/1, Gain4/1, θ_m [rad]/1  "θ_m"
  Gain8/1 -> Integrator3/1  "dT_s/dt"
  Integrator1/1 -> Square/1, Gain6/1, T. Inversa de Park/1(f_q), i_qs [A]/1, 1.5*P_p*λ′m/1  "i_qs"
  Integrator2/1 -> Integrator/1, P_p*λ′m/1, Gain1/1, ω_m [rad/s]/1  "ω_m"
  Add1/1 -> Gain7/1
  Gain/1 -> Integrator4/1, Square1/1  "di_ds/dt"
  Integrator4/1 -> T. Inversa de Park/2(f_d), i_ds [A]/1, Gain/1  "i_ds"
  Square1/1 -> Add4/1
  Add4/1 -> 1.5*R_sREF/1
  P_p/1 -> T. Inversa de Park1/4(θ_r), T. Inversa de Park/4(θ_r)
  T. Inversa de Park/3(f_c) -> I_c [A]/1
  T. Inversa de Park/2(f_b) -> I_b [A]/1
  T. Inversa de Park/1(f_a) -> I_a [A]/1
  Constant/1 -> T. Inversa de Park/3(f_0)
  Constant1/1 -> T. Inversa de Park1/2(f_d)
  Constant2/1 -> T. Inversa de Park1/3(f_0)
  T. Inversa de Park1/1(f_a) -> V_a/1
  T. Inversa de Park1/2(f_b) -> V_b/1
  T. Inversa de Park1/3(f_c) -> V_c/1

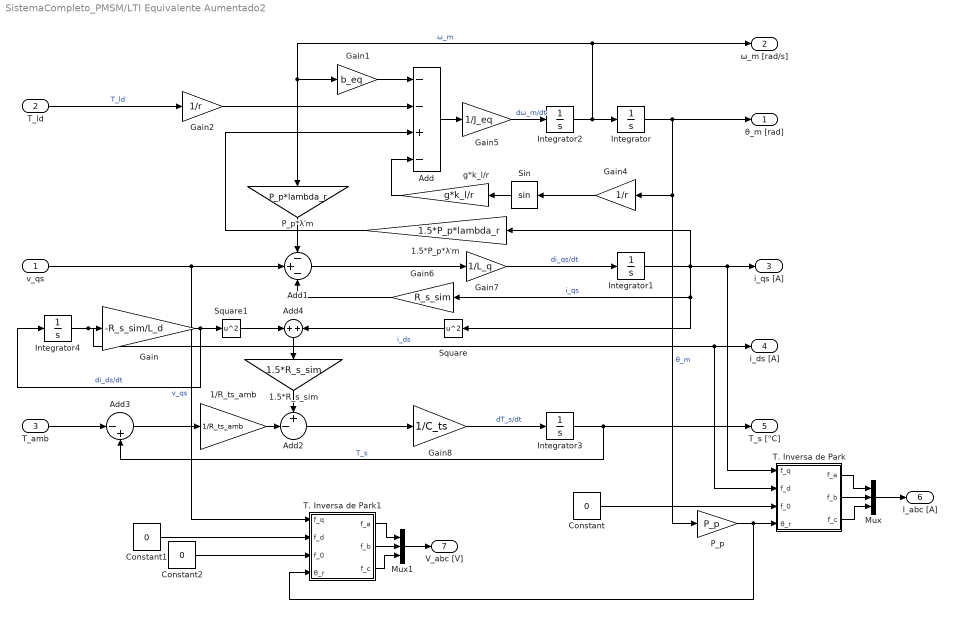
== system SistemaCompleto_PMSM/LTI Equivalente Aumentado2 ==
  v_qs : Inport
  T_ld : Inport  Port=2
  T_amb : Inport  Port=3
  1.5*P_p*λ′m : Gain  Gain=1.5*P_p*lambda_r
  1.5*R_s_sim : Gain  Gain=1.5*R_s_sim
  1/R_ts_amb : Gain  Gain=1/R_ts_amb
  Add : Sum  Inputs=--+-
  Add1 : Sum  Inputs=-+-
  Add2 : Sum  Inputs=+-|
  Add3 : Sum  Inputs=|-+
  Add4 : Sum
  Constant : Constant  Value=0
  Constant1 : Constant  Value=0
  Constant2 : Constant  Value=0
  Gain : Gain  Gain=-R_s_sim/L_d
  Gain1 : Gain  Gain=b_eq
  Gain2 : Gain  Gain=1/r
  Gain4 : Gain  Gain=1/r
  Gain5 : Gain  Gain=1/J_eq
  Gain6 : Gain  Gain=R_s_sim
  Gain7 : Gain  Gain=1/L_q
  Gain8 : Gain  Gain=1/C_ts
  Integrator{,1..2,4} (4 alike) : Integrator
  Integrator3 : Integrator  InitialCondition=T_amb
  Mux : Mux  Inputs=3
  Mux1 : Mux  Inputs=3
  P_p : Gain  Gain=P_p
  P_p*λ′m : Gain  Gain=P_p*lambda_r
  Sin : Trigonometry
  Square : Math  Operator=square
  Square1 : Math  Operator=square
  T. Inversa de Park : Subsystem
  T. Inversa de Park1 : Subsystem
  g*k_l/r : Gain  Gain=g*k_l/r
  θ_m [rad] : Outport
  ω_m [rad/s] : Outport  Port=2
  i_qs [A] : Outport  Port=3
  i_ds [A] : Outport  Port=4
  T_s [°C] : Outport  Port=5
  I_abc [A] : Outport  Port=6
  V_abc [V] : Outport  Port=7
  wires:
  P_p*λ′m/1 -> Add1/1
  Add/1 -> Gain5/1
  T_amb/1 -> Add3/1
  g*k_l/r/1 -> Add/4
  Gain1/1 -> Add/1
  v_qs/1 -> T. Inversa de Park1/1(f_q), Add1/2  "v_qs"
  1.5*P_p*λ′m/1 -> Add/3
  Gain6/1 -> Add1/3
  Gain2/1 -> Add/2
  T_ld/1 -> Gain2/1  "T_ld"
  Sin/1 -> g*k_l/r/1
  1.5*R_s_sim/1 -> Add2/1
  1/R_ts_amb/1 -> Add2/2
  Add2/1 -> Gain8/1
  Square/1 -> Add4/2
  Gain5/1 -> Integrator2/1  "dω_m/dt"
  Gain4/1 -> Sin/1
  Add3/1 -> 1/R_ts_amb/1
  Integrator3/1 -> T_s [°C]/1, Add3/2  "T_s"
  Gain7/1 -> Integrator1/1  "di_qs/dt"
  Integrator/1 -> P_p/1, Gain4/1, θ_m [rad]/1  "θ_m"
  Gain8/1 -> Integrator3/1  "dT_s/dt"
  Integrator1/1 -> Square/1, Gain6/1, T. Inversa de Park/1(f_q), i_qs [A]/1, 1.5*P_p*λ′m/1  "i_qs"
  Integrator2/1 -> Integrator/1, P_p*λ′m/1, Gain1/1, ω_m [rad/s]/1  "ω_m"
  Add1/1 -> Gain7/1
  Gain/1 -> Square1/1, Integrator4/1  "di_ds/dt"
  Integrator4/1 -> T. Inversa de Park/2(f_d), i_ds [A]/1, Gain/1  "i_ds"
  Square1/1 -> Add4/1
  Add4/1 -> 1.5*R_s_sim/1
  P_p/1 -> T. Inversa de Park1/4(θ_r), T. Inversa de Park/4(θ_r)
  T. Inversa de Park/3(f_c) -> Mux/3
  T. Inversa de Park/2(f_b) -> Mux/2
  T. Inversa de Park/1(f_a) -> Mux/1
  Constant/1 -> T. Inversa de Park/3(f_0)
  Constant1/1 -> T. Inversa de Park1/2(f_d)
  Constant2/1 -> T. Inversa de Park1/3(f_0)
  T. Inversa de Park1/1(f_a) -> Mux1/1
  T. Inversa de Park1/2(f_b) -> Mux1/2
  T. Inversa de Park1/3(f_c) -> Mux1/3
  Mux/1 -> I_abc [A]/1
  Mux1/1 -> V_abc [V]/1

== system SistemaCompleto_PMSM/LTI Equivalente Nominal ==
  v_qs : Inport
  T_ld : Inport  Port=2
  T_amb : Inport  Port=3
  1.5*P_p*λ′m : Gain  Gain=1.5*P_p*lambda_r
  1.5*R_sREF : Gain  Gain=1.5*R_sREF
  1/R_ts_amb : Gain  Gain=1/R_ts_amb
  Add : Sum  Inputs=--+-
  Add1 : Sum  Inputs=-+-
  Add2 : Sum  Inputs=+-|
  Add3 : Sum  Inputs=|-+
  Gain1 : Gain  Gain=b_eq
  Gain2 : Gain  Gain=1/r
  Gain4 : Gain  Gain=1/r
  Gain5 : Gain  Gain=1/J_eq
  Gain6 : Gain  Gain=R_sREF
  Gain7 : Gain  Gain=1/L_q
  Gain8 : Gain  Gain=1/C_ts
  Integrator{,1..3} (4 alike) : Integrator
  P_p*λ′m : Gain  Gain=P_p*lambda_r
  Sin : Trigonometry
  Square : Math  Operator=square
  g*k_l/r : Gain  Gain=g*k_l/r
  θ_m : Outport
  ω_m : Outport  Port=2
  i_qs : Outport  Port=3
  T_s : Outport  Port=4
  wires:
  Add1/1 -> Gain7/1
  Integrator2/1 -> ω_m/1, Gain1/1, P_p*λ′m/1, Integrator/1  "ω_m"
  Integrator1/1 -> i_qs/1, 1.5*P_p*λ′m/1, Square/1, Gain6/1  "i_qs"
  Gain8/1 -> Integrator3/1  "dT_s/dt"
  Integrator/1 -> θ_m/1, Gain4/1  "θ_m"
  Gain7/1 -> Integrator1/1  "di_qs/dt"
  Integrator3/1 -> Add3/2, T_s/1  "T_s"
  Add3/1 -> 1/R_ts_amb/1
  Gain4/1 -> Sin/1
  Gain5/1 -> Integrator2/1  "dω_m/dt"
  Square/1 -> 1.5*R_sREF/1
  Add2/1 -> Gain8/1
  1/R_ts_amb/1 -> Add2/2
  1.5*R_sREF/1 -> Add2/1
  Sin/1 -> g*k_l/r/1
  T_ld/1 -> Gain2/1  "T_ld"
  Gain2/1 -> Add/2
  Gain6/1 -> Add1/3
  1.5*P_p*λ′m/1 -> Add/3
  v_qs/1 -> Add1/2  "v_qs"
  Gain1/1 -> Add/1
  g*k_l/r/1 -> Add/4
  T_amb/1 -> Add3/1
  Add/1 -> Gain5/1
  P_p*λ′m/1 -> Add1/1

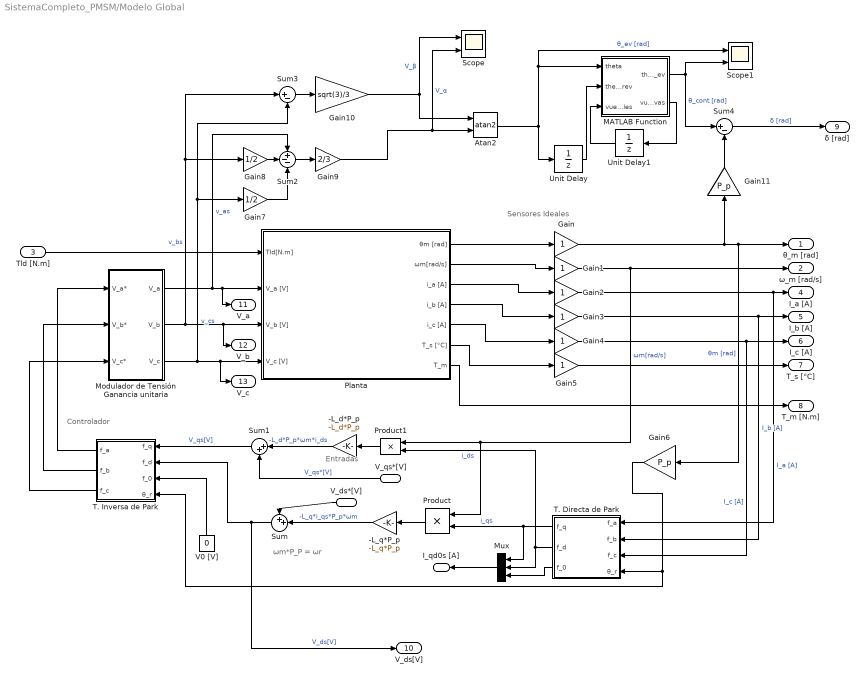
== system SistemaCompleto_PMSM/Modelo Global  ==
  note: ωm*P_P = ωr
  note: Entradas
  note: Sensores Ideales
  note: Controlador
  V_qs*[V] : Inport
  V_ds*[V] : Inport  Port=2
  Tld [N.m] : Inport  Port=3
  -L_d*P_p : Gain  Gain=-L_d*P_p
  -L_q*P_p : Gain  Gain=-L_q*P_p
  Atan2 : Trigonometry  Operator=atan2
  Gain{,1..5} (6 alike) : Gain
  Gain10 : Gain  Gain=sqrt(3)/3
  Gain11 : Gain  Gain=P_p
  Gain6 : Gain  Gain=P_p
  Gain7 : Gain  Gain=1/2
  Gain8 : Gain  Gain=1/2
  Gain9 : Gain  Gain=2/3
  MATLAB Function : MATLAB Function  TreatAsAtomicUnit=on
  Modulador de Tensión Ganancia unitaria : Subsystem
  Mux : Mux  Inputs=3
  Planta : Subsystem
  Product : Product
  Product1 : Product
  Scope : Scope  NumInputPorts=2
  Scope1 : Scope  NumInputPorts=2
  Sum : Sum  Inputs=++|
  Sum1 : Sum  Inputs=|++
  Sum2 : Sum  Inputs=+--
  Sum3 : Sum  Inputs=|+-
  Sum4 : Sum  Inputs=|+-
  T. Directa de Park : Subsystem
  T. Inversa de Park : Subsystem
  Unit Delay : UnitDelay  SampleTime=1e-4  HasFrameUpgradeWarning=on
  Unit Delay1 : UnitDelay  SampleTime=1e-4  HasFrameUpgradeWarning=on
  V0 [V] : Constant  Value=0
  θ_m [rad] : Outport
  ω_m [rad/s] : Outport  Port=2
  I_qd0s [A] : Outport  Port=3
  I_a [A] : Outport  Port=4
  I_b [A] : Outport  Port=5
  I_c [A] : Outport  Port=6
  T_s [°C] : Outport  Port=7
  T_m [N.m] : Outport  Port=8
  δ [rad] : Outport  Port=9
  V_ds[V] : Outport  Port=10
  V_a : Outport  Port=11
  V_b : Outport  Port=12
  V_c : Outport  Port=13
  wires:
  Gain/1 -> Gain6/1, θ_m [rad]/1, Gain11/1  "θm [rad]"
  V0 [V]/1 -> T. Inversa de Park/3(f_0)
  Planta/4(i_b [A]) -> Gain3/1
  Gain4/1 -> T. Directa de Park/3(f_c), I_c [A]/1  "I_c [A]"
  Tld [N.m]/1 -> Planta/1(Tld[N.m])
  Planta/1(θm [rad]) -> Gain/1
  Planta/2(ωm[rad/s]) -> Gain1/1
  Planta/3(i_a [A]) -> Gain2/1
  Planta/5(i_c [A]) -> Gain4/1
  Planta/6(T_s [°C]) -> Gain5/1
  Gain2/1 -> I_a [A]/1, T. Directa de Park/1(f_a)  "I_a [A]"
  Gain5/1 -> T_s [°C]/1
  Gain6/1 -> T. Directa de Park/4(θ_r), T. Inversa de Park/4(θ_r)
  Gain3/1 -> I_b [A]/1, T. Directa de Park/2(f_b)  "I_b [A]"
  Gain1/1 -> ω_m [rad/s]/1, Product1/1, Product/1  "ωm[rad/s]"
  T. Directa de Park/1(f_q) -> Product/2, Mux/1  "i_qs"
  Product/1 -> -L_q*P_p/1
  -L_q*P_p/1 -> Sum/2  "-L_q*i_qs*P_p*ωm"
  V_ds*[V]/1 -> Sum/1
  Sum/1 -> V_ds[V]/1, T. Inversa de Park/2(f_d)  "V_ds[V]"
  Sum1/1 -> T. Inversa de Park/1(f_q)  "V_qs[V]"
  T. Inversa de Park/1(f_a) -> Modulador de Tensión Ganancia unitaria/1(V_a*)
  T. Inversa de Park/2(f_b) -> Modulador de Tensión Ganancia unitaria/2(V_b*)
  T. Inversa de Park/3(f_c) -> Modulador de Tensión Ganancia unitaria/3(V_c*)
  Modulador de Tensión Ganancia unitaria/1(V_a) -> V_a/1, Planta/2(V_a [V]), Sum2/1  "v_as"
  Modulador de Tensión Ganancia unitaria/2(V_b) -> V_b/1, Planta/3(V_b [V]), Sum3/1, Gain8/1  "v_bs"
  Modulador de Tensión Ganancia unitaria/3(V_c) -> V_c/1, Planta/4(V_c [V]), Sum3/2, Gain7/1  "v_cs"
  T. Directa de Park/2(f_d) -> Product1/2, Mux/2  "i_ds"
  Product1/1 -> -L_d*P_p/1
  V_qs*[V]/1 -> Sum1/2  "V_qs*[V]"
  -L_d*P_p/1 -> Sum1/1  "-L_d*P_p*ωm*i_ds"
  T. Directa de Park/3(f_0) -> Mux/3
  Mux/1 -> I_qd0s [A]/1
  Planta/7(T_m) -> T_m [N.m]/1
  Gain7/1 -> Sum2/3
  Gain8/1 -> Sum2/2
  Sum2/1 -> Gain9/1
  Gain9/1 -> Scope/2, Atan2/2  "V_α"
  Sum3/1 -> Gain10/1
  Gain10/1 -> Scope/1, Atan2/1  "V_β"
  Atan2/1 -> Unit Delay/1, MATLAB Function/1(theta), Scope1/1  "θ_ev [rad]"
  Gain11/1 -> Sum4/2
  Sum4/1 -> δ [rad]/1  "δ [rad]"
  MATLAB Function/1(theta_ev) -> Sum4/1, Scope1/2  "θ_cont [rad]"
  MATLAB Function/2(vueltas_nuevas) -> Unit Delay1/1
  Unit Delay1/1 -> MATLAB Function/3(vueltas_actuales)
  Unit Delay/1 -> MATLAB Function/2(theta_prev)

== system SistemaCompleto_PMSM/Modelo Global NL Controlador modulador de torque ==
  note: Controlador
  note: Sensores Ideales
  Tld [N.m] : Inport
  i_ds* : Inport  Port=2
  T_m*[N.m] : Inport  Port=3
  Constant : Constant  Value=1.04
  Desacople de Realimentaciones Fisicas Naturales : Subsystem
  Gain{,1..5} (6 alike) : Gain
  Gain6 : Gain  Gain=P_p
  Modulador de Corriente : Subsystem
  Modulador de Tensión Ganancia unitaria : Subsystem
  Modulador de Torque : Subsystem
  Mux : Mux  Inputs=3
  Planta : Subsystem
  T. Directa de Park : Subsystem
  T. Inversa de Park : Subsystem
  T_neto [N.m] : Scope
  θm(t) [rad] : Outport
  ωm(t) [rad/s] : Outport  Port=2
  I_qd0s [A] : Outport  Port=3
  I_a [A] : Outport  Port=4
  I_b [A] : Outport  Port=5
  I_c [A] : Outport  Port=6
  T_s [°C] : Outport  Port=7
  T_m [N.m] : Outport  Port=8
  T_neto : Outport  Port=9
  wires:
  Gain/1 -> Gain6/1, Modulador de Torque/2(θm [rad]), θm(t) [rad]/1  "θm [rad]"
  Desacople de Realimentaciones Fisicas Naturales/3(v_0s [V]) -> T. Inversa de Park/4(f_0)  "V_0s [V]"
  Planta/4(i_b [A]) -> Gain3/1
  Gain4/1 -> I_c [A]/1, T. Directa de Park/3(f_c)  "I_c [A]"
  Tld [N.m]/1 -> Planta/1(Tld[N.m])
  Planta/1(θm [rad]) -> Gain/1
  Planta/2(ωm[rad/s]) -> Gain1/1
  Planta/3(i_a [A]) -> Gain2/1
  Planta/5(i_c [A]) -> Gain4/1
  Planta/6(T_s [°C]) -> Gain5/1
  Gain2/1 -> T. Directa de Park/1(f_a), I_a [A]/1  "I_a [A]"
  Gain5/1 -> T_s [°C]/1  "T_s [°C]"
  Gain6/1 -> T. Inversa de Park/1(θ_r), T. Directa de Park/4(θ_r)  "θr [rad]"
  Gain3/1 -> I_b [A]/1, T. Directa de Park/2(f_b)  "I_b [A]"
  Gain1/1 -> ωm(t) [rad/s]/1, Modulador de Torque/1(ωm[rad/s]), Desacople de Realimentaciones Fisicas Naturales/2(ωm)  "ωm[rad/s]"
  T. Directa de Park/1(f_q) -> Desacople de Realimentaciones Fisicas Naturales/3(i_qs), Modulador de Corriente/1(i_qs), Mux/1  "i_qs"
  Desacople de Realimentaciones Fisicas Naturales/2(v_ds [V]) -> T. Inversa de Park/3(f_d)  "V_ds[V]"
  Desacople de Realimentaciones Fisicas Naturales/1(v_qs [V]) -> T. Inversa de Park/2(f_q)  "V_qs[V]"
  T. Inversa de Park/1(f_a) -> Modulador de Tensión Ganancia unitaria/3(V_a*)
  T. Inversa de Park/2(f_b) -> Modulador de Tensión Ganancia unitaria/2(V_b*)
  T. Inversa de Park/3(f_c) -> Modulador de Tensión Ganancia unitaria/1(V_c*)
  Modulador de Tensión Ganancia unitaria/1(V_a) -> Planta/2(V_a [V])
  Modulador de Tensión Ganancia unitaria/2(V_b) -> Planta/3(V_b [V])
  Modulador de Tensión Ganancia unitaria/3(V_c) -> Planta/4(V_c [V])
  T. Directa de Park/2(f_d) -> Modulador de Corriente/4(i_ds), Desacople de Realimentaciones Fisicas Naturales/8(i_ds), Modulador de Torque/4(i_ds [A]), Mux/2  "i_ds"
  T. Directa de Park/3(f_0) -> Desacople de Realimentaciones Fisicas Naturales/7(i_0s), Modulador de Corriente/6(i_0s), Modulador de Corriente/5(i_0s*), Mux/3  "i_0s"
  Mux/1 -> I_qd0s [A]/1
  Planta/7(T_m) -> T_m [N.m]/1
  Modulador de Corriente/1(v_qs*) -> Desacople de Realimentaciones Fisicas Naturales/4(v_qs*)
  Modulador de Torque/1(i_qs*) -> Modulador de Corriente/2(i_qs*)
  i_ds*/1 -> Modulador de Corriente/3(i_ds*)
  Modulador de Corriente/2(v_ds*) -> Desacople de Realimentaciones Fisicas Naturales/5(v_ds*)
  Modulador de Corriente/3(v_0s*) -> Desacople de Realimentaciones Fisicas Naturales/6(v_0s*)
  T_m*[N.m]/1 -> Modulador de Torque/3(T_m*'[N.m])
  Planta/8(T_neto) -> T_neto [N.m]/1, T_neto/1  "T_neto [N.m]"
  Planta/9(R_s) -> ?
  Constant/1 -> Desacople de Realimentaciones Fisicas Naturales/1(R_s)

== system SistemaCompleto_PMSM/Modelo Global NL Controlador modulador de torque1 ==
  note: Controlador
  note: Sensores Ideales
  Tld [N.m] : Inport
  i_ds* : Inport  Port=2
  θl*(t) : Inport  Port=3
  Constant : Constant  Value=R_sREF
  Controlador PID de Posicion : Subsystem
  Desacople de Realimentaciones Fisicas Naturales : Subsystem
  Gain{,1..5} (6 alike) : Gain
  Gain6 : Gain  Gain=P_p
  Modulador de Corriente : Subsystem
  Modulador de Tensión Ganancia unitaria : Subsystem
  Modulador de Torque : Subsystem
  Mux : Mux  Inputs=3
  Planta : Subsystem
  Setpoint : Subsystem
  T. Directa de Park : Subsystem
  T. Inversa de Park : Subsystem
  T_neto [N.m] : Scope
  θm(t) [rad] : Outport
  ωm(t) [rad/s] : Outport  Port=2
  I_qd0s [A] : Outport  Port=3
  I_a [A] : Outport  Port=4
  I_b [A] : Outport  Port=5
  I_c [A] : Outport  Port=6
  T_s [°C] : Outport  Port=7
  T_m [N.m] : Outport  Port=8
  T_neto : Outport  Port=9
  θm* [rad] : Outport  Port=10
  wires:
  Gain/1 -> Gain6/1, Modulador de Torque/2(θm [rad]), θm(t) [rad]/1  "θm [rad]"
  Desacople de Realimentaciones Fisicas Naturales/3(v_0s [V]) -> T. Inversa de Park/4(f_0)  "V_0s [V]"
  Planta/4(i_b [A]) -> Gain3/1
  Gain4/1 -> I_c [A]/1, T. Directa de Park/3(f_c)  "I_c [A]"
  Tld [N.m]/1 -> Planta/1(Tld[N.m])
  Planta/1(θm [rad]) -> Gain/1
  Planta/2(ωm[rad/s]) -> Gain1/1
  Planta/3(i_a [A]) -> Gain2/1
  Planta/5(i_c [A]) -> Gain4/1
  Planta/6(T_s [°C]) -> Gain5/1
  Gain2/1 -> T. Directa de Park/1(f_a), I_a [A]/1  "I_a [A]"
  Gain5/1 -> T_s [°C]/1  "T_s [°C]"
  Gain6/1 -> T. Inversa de Park/1(θ_r), T. Directa de Park/4(θ_r)  "θr [rad]"
  Gain3/1 -> I_b [A]/1, T. Directa de Park/2(f_b)  "I_b [A]"
  Gain1/1 -> ωm(t) [rad/s]/1, Controlador PID de Posicion/1(ωm[rad/s]), Modulador de Torque/1(ωm[rad/s]), Desacople de Realimentaciones Fisicas Naturales/2(ωm)  "ωm[rad/s]"
  T. Directa de Park/1(f_q) -> Desacople de Realimentaciones Fisicas Naturales/3(i_qs), Modulador de Corriente/1(i_qs), Mux/1  "i_qs"
  Desacople de Realimentaciones Fisicas Naturales/2(v_ds [V]) -> T. Inversa de Park/3(f_d)  "V_ds[V]"
  Desacople de Realimentaciones Fisicas Naturales/1(v_qs [V]) -> T. Inversa de Park/2(f_q)  "V_qs[V]"
  T. Inversa de Park/1(f_a) -> Modulador de Tensión Ganancia unitaria/3(V_a*)
  T. Inversa de Park/2(f_b) -> Modulador de Tensión Ganancia unitaria/2(V_b*)
  T. Inversa de Park/3(f_c) -> Modulador de Tensión Ganancia unitaria/1(V_c*)
  Modulador de Tensión Ganancia unitaria/1(V_a) -> Planta/2(V_a [V])
  Modulador de Tensión Ganancia unitaria/2(V_b) -> Planta/3(V_b [V])
  Modulador de Tensión Ganancia unitaria/3(V_c) -> Planta/4(V_c [V])
  T. Directa de Park/2(f_d) -> Modulador de Corriente/4(i_ds), Desacople de Realimentaciones Fisicas Naturales/8(i_ds), Modulador de Torque/4(i_ds [A]), Mux/2  "i_ds"
  T. Directa de Park/3(f_0) -> Desacople de Realimentaciones Fisicas Naturales/7(i_0s), Modulador de Corriente/6(i_0s), Modulador de Corriente/5(i_0s*), Mux/3  "i_0s"
  Mux/1 -> I_qd0s [A]/1
  Planta/7(T_m) -> T_m [N.m]/1
  Modulador de Corriente/1(v_qs*) -> Desacople de Realimentaciones Fisicas Naturales/4(v_qs*)
  Modulador de Torque/1(i_qs*) -> Modulador de Corriente/2(i_qs*)
  i_ds*/1 -> Modulador de Corriente/3(i_ds*)
  Modulador de Corriente/2(v_ds*) -> Desacople de Realimentaciones Fisicas Naturales/5(v_ds*)
  Modulador de Corriente/3(v_0s*) -> Desacople de Realimentaciones Fisicas Naturales/6(v_0s*)
  Planta/8(T_neto) -> T_neto [N.m]/1, T_neto/1  "T_neto [N.m]"
  Planta/9(R_s) -> Desacople de Realimentaciones Fisicas Naturales/1(R_s)
  Controlador PID de Posicion/1(Tm*') -> Modulador de Torque/3(T_m*'[N.m])
  θl*(t)/1 -> Setpoint/1(θl*(t))
  Setpoint/1(θm* [rad]) -> θm* [rad]/1
  Setpoint/2(ωm*[rad/s]) -> Controlador PID de Posicion/2(ωm*[rad/s])
